simulink model "Quad_Plant_dynamics"  (R2023b)
settings: Solver=FixedStepAuto  StartTime=0.0  StopTime=10.0  RelTol=1e-3
undefined symbols (not defined in the file): altToPrsBias, altToPrsGain, b, battCapacity, c, contact, dragCoeffMov, fractalcoef, g, mass, ms2_to_mg, ms_to_cms, Payload, rotorDir, rotorPositions, rotorThrustMax, rotorTimeConst, rotorTorqueMax, SampleTime, windVel
libraries: simulink x3, uavmavlinklib x3, sharedtransform x2, robotcorelib x2, sensorinslib x1, shared6dof x1, mspsensorlib x1, uavutilslib x1
(part 2 of 2)

== matlab function Quad_Plant_dynamics/Quadcopter model/Force and Moment Calculation/Rotor Model/Thrust & Torque model/Subsystem/MATLAB Function ==
  settings: updateMethod=DISCRETE
  data: epsilon input; T output; Vinf input; alpha_set input; b input; c input; Q output; omega output
function [T, Q, omega]= BET(epsilon, Vinf, alpha_set, b, c)         
    
    omega=epsilon*837.758041+1e-6; 
    %air density
    rho=1.225;

    %angles
    theta=atan(0.1016./(2.*pi.*b));


    deltaT=zeros(10, length(b));
    deltaQ=deltaT;

%   while isreal(deltaT)==0
        for i=1:length(b)
  
            A= 0;%randi(3000)*0.0001; %initial guess for the axial inflow factor
            B= 0;%randi(3000)*0.0001; %initial guess for the swirl factor
            if i==1 || i==22
                dr=0.5*(b(2)-b(1));
            else
                dr=b(2)-b(1);
            end
            for j=1:10
                V0=Vinf*(1+A);
                V2=omega*b(i)*(1-B);
                V1=sqrt(V0^2+V2^2);
                alpha=atan(V0/V2);
                phi=theta(i)+alpha_set-alpha;
                % Cl=CL(phi);
                % Cd=CD(phi);
                phideg=rad2deg(phi);
                if phideg<=7.7
                    cl=0.1022*phideg+0.3749;
                elseif phideg>7.7 && phideg<=20
                    cl=0.0000118782*phideg^5-0.0006558208*phideg^4+0.0133404539* phideg^3-0.1264259735* phideg^2+0.6181804301*phideg-0.2152921158;
                else %phideg>20
                    cl=1.3805-1.3805*phideg/70;
                end
                alphadata=-8:1:19;
                CDdata=4.*[0.091 0.0838 0.0749 0.06 0.0305 0.028 0.0234 0.02 0.018 0.0174 0.0168 0.018 0.0186 0.0192 0.0197 0.022 0.0234 0.0251 0.0275 0.0317 0.0377 0.0455 0.0604 0.074 0.0868 0.108 0.1437 0.223];
                phideg=rad2deg(phi);
                if phideg>=-8 && phideg<=19
                    dragcoefficient=interp1(alphadata, CDdata, phideg);
                elseif phideg>19
                    dragcoefficient=0.892+(phideg-19)*0.016;
                else %phideg<-8
                    dragcoefficient=0.346+(-phideg-8)*0.02;
                end 
                Cl=cl;
                Cd=dragcoefficient;
                deltaT(j, i)=real(rho*V1^2*c(i)*(Cl*cos(alpha)-Cd*sin(alpha))*dr);
                deltaQ(j, i)=real(rho*V1^2*c(i)*(Cl*sin(alpha)+Cd*cos(alpha))*dr*b(i));
                % S=(pi*(b(i)+0.5*dr)^2)-(pi*(b(i)-0.5*dr)^2);
                % if Vinf~=0
                %     Btemp=deltaQ(j ,i)/(4*pi*b(i)^3*Vinf*(1+A)*omega*dr);
                %     Atemp=(-2*S*rho*Vinf^2+sqrt(4*S^2*rho^2*Vinf^4+8*deltaT(j, i)*S*rho*Vinf^2))/(4*S*rho*Vinf^2);
                % else
                %     Atemp=A;
                %     Btemp=B;
                % 
                % end    
                % A=0.5*(A+Atemp);
                % B=0.5*(B+Btemp);
            end
        end
%         if isreal(deltaT)==1
%             break
%         end
%     end

Ttemp=deltaT(10, :);
Qtemp=deltaQ(10, :);
T=real(sum(Ttemp));
Q=real(sum(Qtemp));
% M=sum(Mtemp);
% prop=T*Vinf/(omega*Q)
% zetashaft(Q, omega)
end

== matlab function Quad_Plant_dynamics/Quadcopter model/Force and Moment Calculation/Aerodynamic drag/calcDragVector ==
  data: airVel input; dragVec output; dragCoeff input
function dragVec = fcn(airVel, dragCoeff)

dragVec = dragCoeff * airVel .* airVel;
% dragVec(3)=0;
end

== matlab function Quad_Plant_dynamics/Quadcopter model/Force and Moment Calculation/Rotor Model/Thrust & Torque model/Subsystem/MATLAB Function2 ==
  data: vx input; Vinf output; vy input; vz input; phi input; theta input
function Vinf = inflowSpeed(vx, vy, vz, phi, theta)
    vxContribution=vx*sin(theta);
    vyContribution=vy*sin(phi);
    vzContribution=vz*cos(theta)*cos(phi);
    Vinf=sqrt(vxContribution^2+vyContribution^2+vzContribution^2);

== matlab function Quad_Plant_dynamics/Quadcopter model/Force and Moment Calculation/Rotor Model/MATLAB Function ==
  data: thrustEachRotor input; tauEachRotor input; rotorPositions input; netF output; netM output; rotorDir input; phi input; theta input
function [netF, netM] = getForceMoment(thrustEachRotor, tauEachRotor, rotorPositions, rotorDir, phi, theta)
%#codegen
Fx = sum(thrustEachRotor)*-sin(theta);
Fy = sum(thrustEachRotor)*-sin(phi);
Fz = -sum(thrustEachRotor)*cos(theta)*cos(phi);

netF = [Fx; Fy; Fz];

netM = [0; 0; 0]; %initialize
    for i = 1:4
        rotPos = rotorPositions(:, i);
        Fi = [0, 0, -thrustEachRotor(i)]';
        netM = netM +  cross(rotPos, Fi);%contribution from thrusts of each propeller
        netM(3) = netM(3) - rotorDir(i)*tauEachRotor(i); %contribution from counter torque acting on propeller
    end

end

== matlab function Quad_Plant_dynamics/Quadcopter model/Force and Moment Calculation/Rotor Model/Thrust & Torque model/Subsystem1/MATLAB Function ==
  settings: updateMethod=DISCRETE
  data: epsilon input; T output; Vinf input; alpha_set input; b input; c input; Q output; omega output
function [T, Q, omega]= BET(epsilon, Vinf, alpha_set, b, c)         
    
    omega=epsilon*837.758041+1e-6; 
    %air density
    rho=1.225;

    %angles
    theta=atan(0.1016./(2.*pi.*b));


    deltaT=zeros(10, length(b));
    deltaQ=deltaT;

%   while isreal(deltaT)==0
        for i=1:length(b)
  
            A= 0;%randi(3000)*0.0001; %initial guess for the axial inflow factor
            B= 0;%randi(3000)*0.0001; %initial guess for the swirl factor
            if i==1 || i==22
                dr=0.5*(b(2)-b(1));
            else
                dr=b(2)-b(1);
            end
            for j=1:10
                V0=Vinf*(1+A);
                V2=omega*b(i)*(1-B);
                V1=sqrt(V0^2+V2^2);
                alpha=atan(V0/V2);
                phi=theta(i)+alpha_set-alpha;
                % Cl=CL(phi);
                % Cd=CD(phi);
                phideg=rad2deg(phi);
                if phideg<=7.7
                    cl=0.1022*phideg+0.3749;
                elseif phideg>7.7 && phideg<=20
                    cl=0.0000118782*phideg^5-0.0006558208*phideg^4+0.0133404539* phideg^3-0.1264259735* phideg^2+0.6181804301*phideg-0.2152921158;
                else %phideg>20
                    cl=1.3805-1.3805*phideg/70;
                end
                alphadata=-8:1:19;
                CDdata=4.*[0.091 0.0838 0.0749 0.06 0.0305 0.028 0.0234 0.02 0.018 0.0174 0.0168 0.018 0.0186 0.0192 0.0197 0.022 0.0234 0.0251 0.0275 0.0317 0.0377 0.0455 0.0604 0.074 0.0868 0.108 0.1437 0.223];
                phideg=rad2deg(phi);
                if phideg>=-8 && phideg<=19
                    dragcoefficient=interp1(alphadata, CDdata, phideg);
                elseif phideg>19
                    dragcoefficient=0.892+(phideg-19)*0.016;
                else %phideg<-8
                    dragcoefficient=0.346+(-phideg-8)*0.02;
                end 
                Cl=cl;
                Cd=dragcoefficient;
                deltaT(j, i)=real(rho*V1^2*c(i)*(Cl*cos(alpha)-Cd*sin(alpha))*dr);
                deltaQ(j, i)=real(rho*V1^2*c(i)*(Cl*sin(alpha)+Cd*cos(alpha))*dr*b(i));
                % S=(pi*(b(i)+0.5*dr)^2)-(pi*(b(i)-0.5*dr)^2);
                % if Vinf~=0
                %     Btemp=deltaQ(j ,i)/(4*pi*b(i)^3*Vinf*(1+A)*omega*dr);
                %     Atemp=(-2*S*rho*Vinf^2+sqrt(4*S^2*rho^2*Vinf^4+8*deltaT(j, i)*S*rho*Vinf^2))/(4*S*rho*Vinf^2);
                % else
                %     Atemp=A;
                %     Btemp=B;
                % 
                % end    
                % A=0.5*(A+Atemp);
                % B=0.5*(B+Btemp);
            end
        end
%         if isreal(deltaT)==1
%             break
%         end
%     end

Ttemp=deltaT(10, :);
Qtemp=deltaQ(10, :);
T=real(sum(Ttemp));
Q=real(sum(Qtemp));
% M=sum(Mtemp);
% prop=T*Vinf/(omega*Q)
% zetashaft(Q, omega)
end

== matlab function Quad_Plant_dynamics/Quadcopter model/Force and Moment Calculation/Rotor Model/Thrust & Torque model/Subsystem1/MATLAB Function1 ==
  data: Q input; shaftefficiency output; omega input
function shaftefficiency=zetashaft(Q, omega)
    Kv=880;
    Kv=Kv*2*pi/60;
    Kt=1/Kv;
    R=0.108;
    Id=0.8; %drain current
    Vd=R*Id; %drain voltage
    VRPM=omega/Kv;
    I=Q/Kt;
    Vr=I*R;
    shaftefficiency=Q*omega/((VRPM+Vr+Vd)*(I+Id));
end

== matlab function Quad_Plant_dynamics/Quadcopter model/Force and Moment Calculation/Rotor Model/Thrust & Torque model/Subsystem1/MATLAB Function2 ==
  data: vx input; Vinf output; vy input; vz input; phi input; theta input
function Vinf = inflowSpeed(vx, vy, vz, phi, theta)
    vxContribution=vx*sin(theta);
    vyContribution=vy*sin(phi);
    vzContribution=vz*cos(theta)*cos(phi);
    Vinf=sqrt(vxContribution^2+vyContribution^2+vzContribution^2);
